simulink model "OutputToVisualization"  (R2016b)
settings: Solver=FixedStepDiscrete  StartTime=0.0  StopTime=10.0  FixedStep=sCoreParams.core.stepPeriod  RelTol=1e-3  EnableMultiTasking=on
undefined symbols (not defined in the file or in its folder): sCoreParams, sCoreParams_viz_channelInds, sCoreParams_viz_featureInds
libraries: simulink x2, xpcrtudplib x2, xpcutilitieslib x1, xpcobsoletelib x1
settings Model: DataTypeOverride=Double  MinMaxOverflowLogging=ForceOff  Creator=rzelmann  LastModifiedBy=rzelmann
settings SolverCC: EnableConcurrentExecution=on  ConcurrentTasks=on  AutoInsertRateTranBlk=on
settings DataIOCC: SaveFormat=StructureWithTime  SaveOutput=off  SignalLogging=off  DSMLogging=off  SaveTime=off
settings OptimizationCC: BlockReduction=off  DefaultParameterBehavior=Inlined  LifeSpan=inf
settings DebuggingCC: AllowSymbolicDim=off  SFUnexpectedBacktrackingDiag=warning  SFNoUnconditionalDefaultTransitionDiag=warning  SFExecutionAtInitializationDiag=none
settings HardwareCC: ProdBitPerPointer=32  ProdBitPerSizeT=32  ProdBitPerPtrDiffT=32  ProdLargestAtomicFloat=None  ProdWordSize=32  ProdLongLongMode=on  ProdHWDeviceType=Generic->32-bit x86 compatible
settings ModelReferenceCC: UpdateModelReferenceTargets=Force  ParallelModelReferenceMATLABWorkerInit=Load Top Model  ModelReferenceNumInstancesAllowed=Single  ModelReferencePassRootInputsByReference=off
settings RTWCC: SystemTargetFile=slrt.tlc  TemplateMakefile=slrt_default_tmf  Description=Simulink Real-Time  RTWCompilerOptimization=on
settings CodeAppCC: MaxIdLength=63
settings TargetCC: CodeReplacementLibrary=XPC_BLAS  ParMdlRefBuildCompliant=on  ConcurrentExecutionCompliant=on  GeneratePreprocessorConditionals=Use local settings  MatFileLogging=on  MATLABClassNameForMDSCustomization=xpcAperiodicCustomization
settings ConfigComp: CovMetricSettings=dw  CovHtmlReporting=on  CovSaveCumulativeToWorkspaceVar=on  CovSaveSingleToWorkspaceVar=on  CovExternalEMLEnable=off

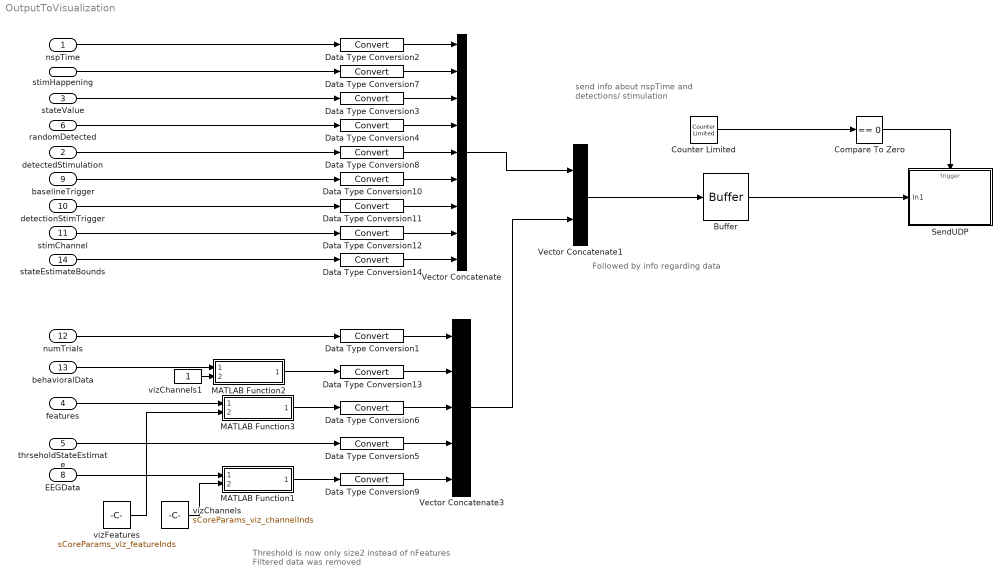
== system OutputToVisualization ==
  note: Threshold is now only size2 instead of nFeatures
      | Filtered data was removed
  note: Followed by info regarding data
  note: send info about nspTime
      |  and detections/ stimulation
  nspTime : Inport  SampleTime=sCoreParams.core.stepPeriod
  detectedStimulation : Inport  Port=2  OutDataTypeStr=boolean  SampleTime=sCoreParams.core.stepPeriod
  stateValue : Inport  Port=3  OutDataTypeStr=double  SampleTime=sCoreParams.core.stepPeriod
  features : Inport  Port=4  PortDimensions=[1 sCoreParams.viz.nFeatures]  SampleTime=sCoreParams.core.stepPeriod
  thrseholdStateEstimate : Inport  Port=5  PortDimensions=2  SampleTime=sCoreParams.core.stepPeriod
  randomDetected : Inport  Port=6  OutDataTypeStr=boolean  SampleTime=sCoreParams.core.stepPeriod
  stimHappening : Inport  Port=7  OutDataTypeStr=boolean  SampleTime=sCoreParams.core.stepPeriod
  EEGData : Inport  Port=8  PortDimensions=[sCoreParams.FrameSize sCoreParams.viz.nChannels]  SampleTime=sCoreParams.core.stepPeriod
  baselineTrigger : Inport  Port=9  OutDataTypeStr=int32  SampleTime=sCoreParams.core.stepPeriod  Interpolate=off
  detectionStimTrigger : Inport  Port=10  OutDataTypeStr=int32  SampleTime=sCoreParams.core.stepPeriod  Interpolate=off
  stimChannel : Inport  Port=11  OutDataTypeStr=int32  PortDimensions=[1 2]  SampleTime=sCoreParams.core.stepPeriod  Interpolate=off
  numTrials : Inport  Port=12  SampleTime=sCoreParams.core.stepPeriod
  behavioralData : Inport  Port=13  PortDimensions=[2 1]  SampleTime=sCoreParams.core.stepPeriod  Interpolate=off
  stateEstimateBounds : Inport  Port=14  OutDataTypeStr=double  PortDimensions=[1 2]  SampleTime=sCoreParams.core.stepPeriod
  Buffer : Buffer  N=sCoreParams.write.broadcastSamp  V=sCoreParams.write.broadcastSamp-1  TreatMby1Signals=One channel  OutputFrames=off
  Compare To Zero : simulink/Logic and Bit Operations/Compare To Zero  relop===  OutDataTypeStr=boolean
  Counter Limited : simulink/Sources/Counter Limited  uplimit=sCoreParams.write.broadcastSamp -1  tsamp=sCoreParams.core.stepPeriod
  Data Type Conversion{1..14} (14 alike) : DataTypeConversion
  MATLAB Function1 : MATLAB Function  TreatAsAtomicUnit=on
  MATLAB Function2 : MATLAB Function  TreatAsAtomicUnit=on
  MATLAB Function3 : MATLAB Function  TreatAsAtomicUnit=on
  SendUDP : Subsystem
  Vector Concatenate : Concatenate  NumInputs=9
  Vector Concatenate1 : Concatenate
  Vector Concatenate3 : Concatenate  NumInputs=5
  vizChannels : Constant  Value=sCoreParams_viz_channelInds
  vizChannels1 : Constant
  vizFeatures : Constant  Value=sCoreParams_viz_featureInds
  wires:
  features/1 -> MATLAB Function3/1(signalIn)
  Data Type Conversion2/1 -> Vector Concatenate/1
  Counter Limited/1 -> Compare To Zero/1
  Compare To Zero/1 -> SendUDP/Trigger
  MATLAB Function3/1(signalOut) -> Data Type Conversion6/1
  Data Type Conversion8/1 -> Vector Concatenate/5
  Vector Concatenate/1 -> Vector Concatenate1/1
  Data Type Conversion7/1 -> Vector Concatenate/2
  Data Type Conversion3/1 -> Vector Concatenate/3
  Data Type Conversion4/1 -> Vector Concatenate/4
  vizChannels/1 -> MATLAB Function1/2(selectCh)
  Vector Concatenate3/1 -> Vector Concatenate1/2
  EEGData/1 -> MATLAB Function1/1(signalIn)
  MATLAB Function1/1(signalOut) -> Data Type Conversion9/1
  Buffer/1 -> SendUDP/1(In1)
  Vector Concatenate1/1 -> Buffer/1
  vizFeatures/1 -> MATLAB Function3/2(selectCh)
  Data Type Conversion10/1 -> Vector Concatenate/6
  Data Type Conversion11/1 -> Vector Concatenate/7
  stimChannel/1 -> Data Type Conversion12/1
  Data Type Conversion12/1 -> Vector Concatenate/8
  nspTime/1 -> Data Type Conversion2/1
  stimHappening/1 -> Data Type Conversion7/1
  stateValue/1 -> Data Type Conversion3/1
  randomDetected/1 -> Data Type Conversion4/1
  detectedStimulation/1 -> Data Type Conversion8/1
  baselineTrigger/1 -> Data Type Conversion10/1
  detectionStimTrigger/1 -> Data Type Conversion11/1
  thrseholdStateEstimate/1 -> Data Type Conversion5/1
  numTrials/1 -> Data Type Conversion1/1
  Data Type Conversion1/1 -> Vector Concatenate3/1
  Data Type Conversion13/1 -> Vector Concatenate3/2
  Data Type Conversion6/1 -> Vector Concatenate3/3
  Data Type Conversion5/1 -> Vector Concatenate3/4
  Data Type Conversion9/1 -> Vector Concatenate3/5
  MATLAB Function2/1(signalOut) -> Data Type Conversion13/1
  behavioralData/1 -> MATLAB Function2/1(signalIn)
  vizChannels1/1 -> MATLAB Function2/2(selectCh)
  stateEstimateBounds/1 -> Data Type Conversion14/1
  Data Type Conversion14/1 -> Vector Concatenate/9

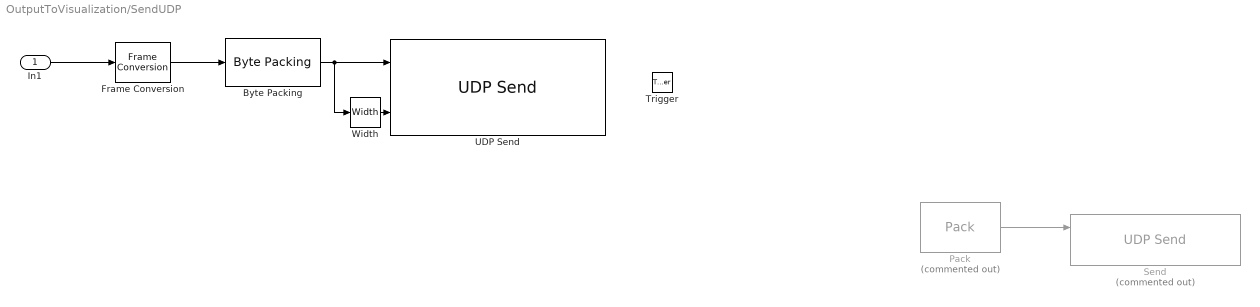
== system OutputToVisualization/SendUDP ==
  In1 : Inport
  Trigger : TriggerPort  VariantControl=Variant  PortDimensions=1
  "Byte Packing " : xpcutilitieslib/Byte Packing   MaskPackedDataType=uint8  MaskUnpackedDataTypes={'double'}  MaskAlignment=1
  Frame Conversion : FrameConversion  InheritSamplingMode=off  OutFrame=Sample-based
  Pack : xpcobsoletelib/Utilities/Pack   Commented=on  datatypes={'double'}  byteAlign=1
  Send : xpcrtudplib/UDP Send  Commented=on  ipAddressVal=Use host-target connection  localPort=59121  toAddress=255.255.255.255  toPort=59123  sampleTime=-1
  UDP Send : xpcrtudplib/UDP Send  ipAddressVal=Use host-target connection  localPort=59121  toAddress=255.255.255.255  toPort=59123  sampleTime=-1
  Width : Width
  wires:
  "Byte Packing "/1 -> Width/1, UDP Send/1
  In1/1 -> Frame Conversion/1
  Frame Conversion/1 -> "Byte Packing "/1
  Pack/1 -> Send/1
  Width/1 -> UDP Send/2

== matlab function OutputToVisualization/MATLAB Function1 ==
  data: signalIn input; signalOut output size=[1 length(sCoreParams_viz_channelInds)]; selectCh input
function signalOut = selectChannelsFromFrame(signalIn,selectCh)
%#codegen
signalOut = signalIn(end,selectCh); %Only send first time point of frame
%signalOut = selectChannelsFromFrame_EML(signalIn,selectCh);

== matlab function OutputToVisualization/MATLAB Function2 ==
  data: signalIn input; signalOut output size=[1 1]; selectCh input
function signalOut = selectChannelsFromFrame(signalIn,selectCh)
%#codegen
signalOut = signalIn(end,selectCh); %Only send first time point of frame
%signalOut = selectChannelsFromFrame_EML(signalIn,selectCh);

== matlab function OutputToVisualization/MATLAB Function3 ==
  data: signalIn input; signalOut output size=[1 length(sCoreParams_viz_featureInds)]; selectCh input
function signalOut = selectChannels(signalIn,selectCh)
%#codegen
signalOut = signalIn(:,selectCh);
%signalOut = selectChannels_EML(signalIn,selectCh);
